simulink model "feedback_control_w_sine"  (R2021b)
settings: Solver=VariableStepAuto  StartTime=0.0  StopTime=50  RelTol=1e-3
undefined symbols (not defined in the file): Ts
libraries: cstblocks x1
settings Model: Creator=varunsampat  LastModifiedBy=varunsampat

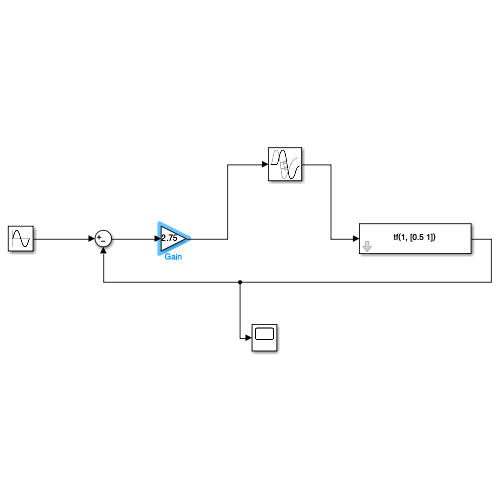
[thumbnail: Simulink's stored preview of the top-level diagram]
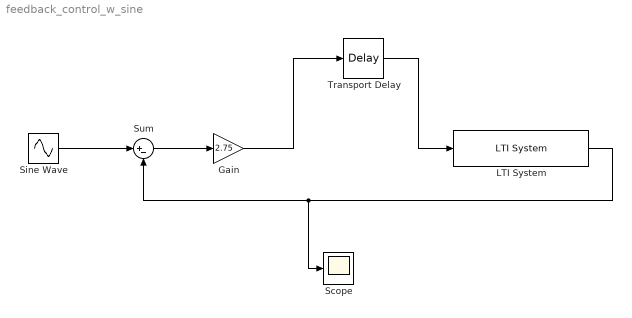
== system feedback_control_w_sine ==
  Gain : Gain  Gain=2.75
  LTI System : cstblocks/LTI System  sys=tf(1, [0.5 1])  IC=[]
  Scope : Scope
  Sine Wave : Sin  SampleTime=0
  Sum : Sum  Inputs=|+-
  Transport Delay : TransportDelay  DelayTime=Ts/2
  wires:
  Sum/1 -> Gain/1
  Sine Wave/1 -> Sum/1
  LTI System/1 -> Scope/1, Sum/2
  Gain/1 -> Transport Delay/1
  Transport Delay/1 -> LTI System/1
